simulink model "Simulink2"  (R2020b)
settings: Solver=VariableStepAuto  StartTime=0.0  StopTime=10  RelTol=1e-3
values from neighbouring files (symbols this model uses):
  Bm = 1.02*10^-9    (= 1.02e-09)    [AugmentedPlant.m]    (also in HW01_Ali_Mohamed_Ali_Hassan_Ali.m = 8.4829584668e-10; Main.m = 8.4829584668e-10)
  C_Optimal = tf(C)    [HW01_Ali_Mohamed_Ali_Hassan_Ali.m]    (also in Main.m)
  C_Optimal_Mixed = tf(C)    [HW01_Ali_Mohamed_Ali_Hassan_Ali.m]    (also in Main.m)
  Jm = 9.5*10^-10    (= 9.5e-10)    [AugmentedPlant.m]    (also in HW01_Ali_Mohamed_Ali_Hassan_Ali.m = 5.4e-08; Main.m = 5.4e-08)
  Ke = 0.378*10^-4    (= 3.78e-05)    [HW01_Ali_Mohamed_Ali_Hassan_Ali.m]    (also in Main.m)
  Km = 3.61*10^-3    (= 0.00361)    [HW01_Ali_Mohamed_Ali_Hassan_Ali.m]    (also in Main.m)
  La = 134*10^-6    (= 0.000134)    [AugmentedPlant.m]    (also in HW01_Ali_Mohamed_Ali_Hassan_Ali.m; Main.m)
  R = 4.36    [HW01_Ali_Mohamed_Ali_Hassan_Ali.m]    (also in Main.m)
libraries: cstblocks x2
settings Model: Creator=15DK0051NL  LastModifiedBy=15DK0051NL

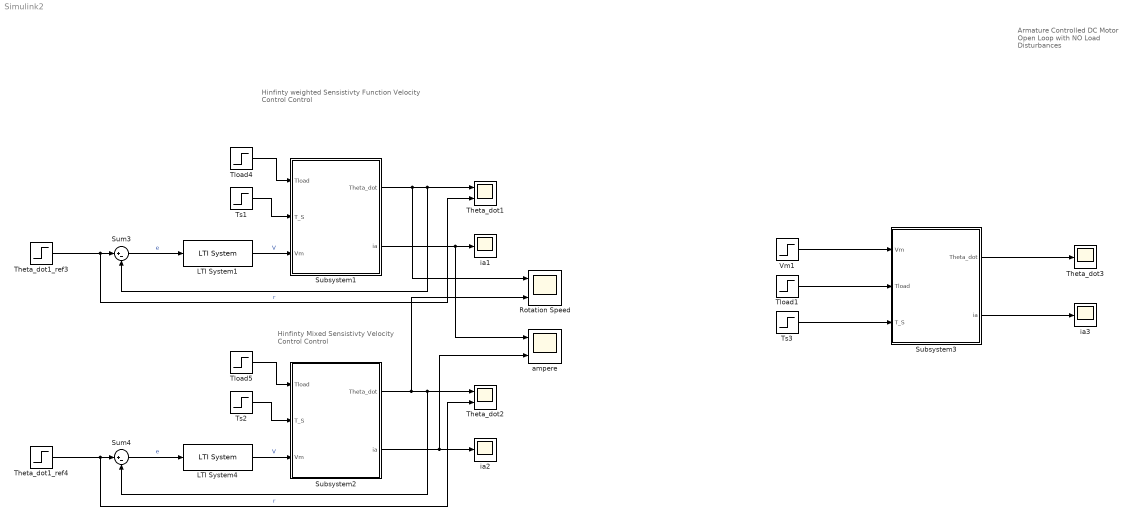
== system Simulink2 ==
  note: Armature Controlled DC Motor
      | Open Loop with NO Load Disturbances
  note: Hinfinty Mixed Sensistivty Velocity Control
      | Control
  note: Hinfinty weighted Sensistivty Function Velocity Control
      | Control
  LTI System1 : cstblocks/LTI System  sys=tf(C_Optimal)  IC=[]
  LTI System4 : cstblocks/LTI System  sys=tf(C_Optimal_Mixed)  IC=[]
  Rotation Speed : Scope  NumInputPorts=2
  Subsystem1 : Subsystem
  Subsystem2 : Subsystem
  Subsystem3 : Subsystem
  Sum3 : Sum  Inputs=|+-
  Sum4 : Sum  Inputs=|+-
  Theta_dot1 : Scope  NumInputPorts=2
  Theta_dot1_ref3 : Step  Time=0  After=20000  SampleTime=0
  Theta_dot1_ref4 : Step  Time=0  After=20000  SampleTime=0
  Theta_dot2 : Scope  NumInputPorts=2
  Theta_dot3 : Scope
  Tload1 : Step  Time=0  After=2.62*10^-3  SampleTime=0
  Tload4 : Step  Time=0  After=2.36*10^-3  SampleTime=0
  Tload5 : Step  Time=0  After=2.6*10^-3  SampleTime=0
  Ts1 : Step  Time=0  After=6.7*10^-3  SampleTime=0
  Ts2 : Step  Time=0  After=6.7*10^-3  SampleTime=0
  Ts3 : Step  Time=0  After=0  SampleTime=0
  Vm1 : Step  Time=0  After=12  SampleTime=0
  ampere : Scope  NumInputPorts=2
  ia1 : Scope
  ia2 : Scope
  ia3 : Scope
  wires:
  Subsystem1/1(Theta_dot) -> Rotation Speed/1, Sum3/2, Theta_dot1/1
  Sum3/1 -> LTI System1/1  "e"
  Theta_dot1_ref3/1 -> Theta_dot1/2, Sum3/1  "r"
  Subsystem1/2(ia) -> ampere/1, ia1/1
  Ts1/1 -> Subsystem1/2(T_S)
  LTI System1/1 -> Subsystem1/3(Vm)  "V"
  Tload4/1 -> Subsystem1/1(Tload)
  Vm1/1 -> Subsystem3/1(Vm)
  Ts3/1 -> Subsystem3/3(T_S)
  Tload1/1 -> Subsystem3/2(Tload)
  Subsystem3/1(Theta_dot) -> Theta_dot3/1
  Subsystem3/2(ia) -> ia3/1
  Ts2/1 -> Subsystem2/2(T_S)
  Theta_dot1_ref4/1 -> Theta_dot2/2, Sum4/1  "r"
  Subsystem2/1(Theta_dot) -> Rotation Speed/2, Sum4/2, Theta_dot2/1
  Tload5/1 -> Subsystem2/1(Tload)
  Sum4/1 -> LTI System4/1  "e"
  Subsystem2/2(ia) -> ampere/2, ia2/1
  LTI System4/1 -> Subsystem2/3(Vm)  "V"

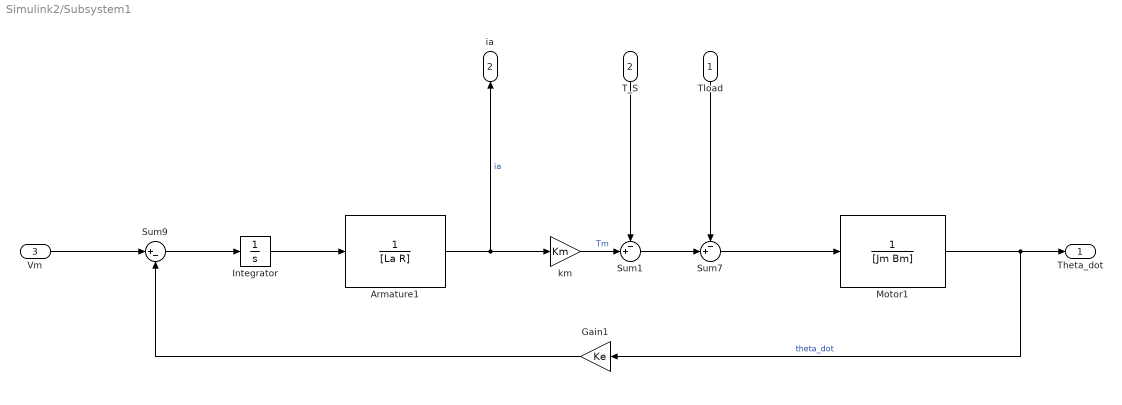
== system Simulink2/Subsystem1 ==
  Tload : Inport
  T_S : Inport  Port=2
  Vm : Inport  Port=3
  Armature1 : TransferFcn  Denominator=[La R]
  Gain1 : Gain  Gain=Ke
  Integrator : Integrator
  Motor1 : TransferFcn  Denominator=[Jm Bm]
  Sum1 : Sum  Inputs=-+|
  Sum7 : Sum  Inputs=-+|
  Sum9 : Sum  Inputs=|+-
  km : Gain  Gain=Km
  Theta_dot : Outport
  ia : Outport  Port=2
  wires:
  Gain1/1 -> Sum9/2
  Armature1/1 -> km/1, ia/1  "ia"
  Motor1/1 -> Theta_dot/1, Gain1/1  "theta_dot"
  Vm/1 -> Sum9/1
  Tload/1 -> Sum7/1
  Sum7/1 -> Motor1/1
  Sum1/1 -> Sum7/2
  km/1 -> Sum1/2  "Tm"
  T_S/1 -> Sum1/1
  Sum9/1 -> Integrator/1
  Integrator/1 -> Armature1/1

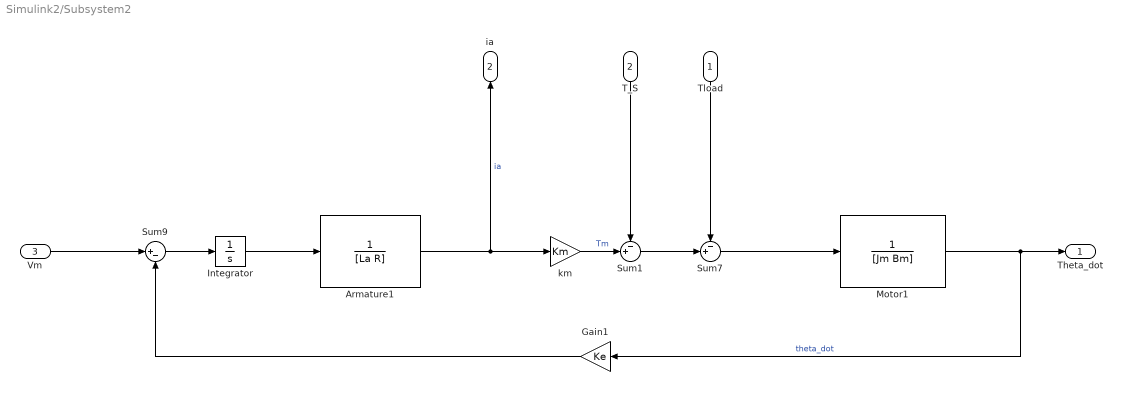
== system Simulink2/Subsystem2 ==
  Tload : Inport
  T_S : Inport  Port=2
  Vm : Inport  Port=3
  Armature1 : TransferFcn  Denominator=[La R]
  Gain1 : Gain  Gain=Ke
  Integrator : Integrator
  Motor1 : TransferFcn  Denominator=[Jm Bm]
  Sum1 : Sum  Inputs=-+|
  Sum7 : Sum  Inputs=-+|
  Sum9 : Sum  Inputs=|+-
  km : Gain  Gain=Km
  Theta_dot : Outport
  ia : Outport  Port=2
  wires:
  Gain1/1 -> Sum9/2
  Armature1/1 -> km/1, ia/1  "ia"
  Motor1/1 -> Theta_dot/1, Gain1/1  "theta_dot"
  Vm/1 -> Sum9/1
  Tload/1 -> Sum7/1
  Sum7/1 -> Motor1/1
  Sum1/1 -> Sum7/2
  km/1 -> Sum1/2  "Tm"
  T_S/1 -> Sum1/1
  Sum9/1 -> Integrator/1
  Integrator/1 -> Armature1/1

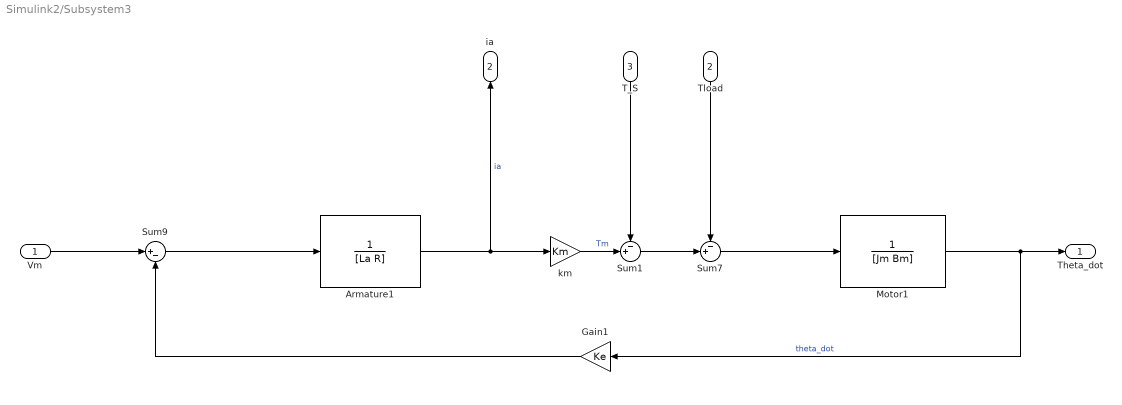
== system Simulink2/Subsystem3 ==
  Vm : Inport
  Tload : Inport  Port=2
  T_S : Inport  Port=3
  Armature1 : TransferFcn  Denominator=[La R]
  Gain1 : Gain  Gain=Ke
  Motor1 : TransferFcn  Denominator=[Jm Bm]
  Sum1 : Sum  Inputs=-+|
  Sum7 : Sum  Inputs=-+|
  Sum9 : Sum  Inputs=|+-
  km : Gain  Gain=Km
  Theta_dot : Outport
  ia : Outport  Port=2
  wires:
  Sum9/1 -> Armature1/1
  Gain1/1 -> Sum9/2
  Armature1/1 -> km/1, ia/1  "ia"
  Motor1/1 -> Theta_dot/1, Gain1/1  "theta_dot"
  Vm/1 -> Sum9/1
  Tload/1 -> Sum7/1
  Sum7/1 -> Motor1/1
  Sum1/1 -> Sum7/2
  km/1 -> Sum1/2  "Tm"
  T_S/1 -> Sum1/1
